simulink model "q5_LQR_sim"  (R2019a)
settings: Solver=VariableStepAuto  StartTime=0.0  StopTime=T  RelTol=1e-3
values from neighbouring files (symbols this model uses):
  A = [0 0 0 1 0 0 ... (first row only)    [q5_LQR_and_H_infinty.m]
  B = [B1, B2]    [q5_LQR_and_H_infinty.m]
  C = [0 0 1 0 0 0]    [q5_LQR_and_H_infinty.m]
undefined symbols (not defined in the file or in its folder): K
settings Model: Creator=ronil  LastModifiedBy=ronil

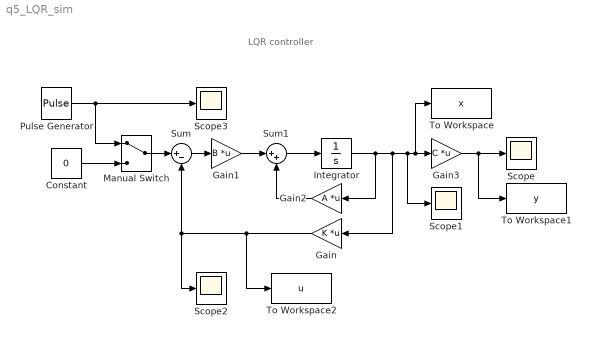
== system q5_LQR_sim ==
  note: LQR controller
  Constant : Constant  Value=0
  Gain : Gain  Gain=K  Multiplication=Matrix(K*u)
  Gain1 : Gain  Gain=B  Multiplication=Matrix(K*u)
  Gain2 : Gain  Gain=A  Multiplication=Matrix(K*u)
  Gain3 : Gain  Gain=C  Multiplication=Matrix(K*u)
  Integrator : Integrator  InitialCondition=[0 0 0 0 0 0]
  Manual Switch : ManualSwitch
  Pulse Generator : DiscretePulseGenerator  PulseType=Time based  Amplitude=30  Period=5  PulseWidth=5
  Scope{,1..3} (4 alike) : Scope
  Sum : Sum  Inputs=|+-
  Sum1 : Sum  Inputs=|++
  To Workspace : ToWorkspace  VariableName=x  SaveFormat=Timeseries  SampleTime=-1
  To Workspace1 : ToWorkspace  VariableName=y  SaveFormat=Timeseries  SampleTime=-1
  To Workspace2 : ToWorkspace  VariableName=u  SaveFormat=Timeseries  SampleTime=-1
  wires:
  Gain/1 -> To Workspace2/1, Scope2/1, Sum/2
  Sum/1 -> Gain1/1
  Gain1/1 -> Sum1/1
  Gain2/1 -> Sum1/2
  Sum1/1 -> Integrator/1
  Integrator/1 -> Gain/1, Scope1/1, To Workspace/1, Gain3/1, Gain2/1
  Gain3/1 -> To Workspace1/1, Scope/1
  Pulse Generator/1 -> Manual Switch/1, Scope3/1
  Manual Switch/1 -> Sum/1
  Constant/1 -> Manual Switch/2
